simulink model "Closed_loop_DC_motor_speed_control"  (R2024a)
settings: Solver=FixedStepAuto  StartTime=0.0  StopTime=3  RelTol=1e-3
values from neighbouring files (symbols this model uses):
  J = 0.00252    [DC_motor_setting.m]
  Kac = 1 / Kpc    (= 0.066209727553)    [DC_motor_setting.m]
  Kas = 1 / Kps    (= 0.0948585204168)    [DC_motor_setting.m]
  Kic = Ra * wcc    (= 2309.95024633)    [DC_motor_setting.m]
  Kis = Kps * wcs / 5    (= 3746.38945888)    [DC_motor_setting.m]
  Kpc = La * wcc    (= 15.1035208414)    [DC_motor_setting.m]
  Kps = J * wcs / Kt    (= 10.5420155786)    [DC_motor_setting.m]
  Kt = Te_rated / Ia_rated    (= 0.424752712124)    [DC_motor_setting.m]
  La = 1.7e-3    (= 0.0017)    [DC_motor_setting.m]
  Ra = 0.26    [DC_motor_setting.m]
  Te_rated = power_rated / wm_rated    (= 10.6188178031)    [DC_motor_setting.m]
  TL = 1    [DC_motor_setting.m]
  Tsw = 1 / fsw    (= 5e-05)    [DC_motor_setting.m]
  Va_rated = 140    [DC_motor_setting.m]
  Vdc = 200    [DC_motor_setting.m]
libraries: spsDCMachineLib x1, spsDCVoltageSourceLib x1, simulink x1, spsUniversalBridgeLib x1, sps_lib x1
settings Model: Creator=d  LastModifiedBy=d

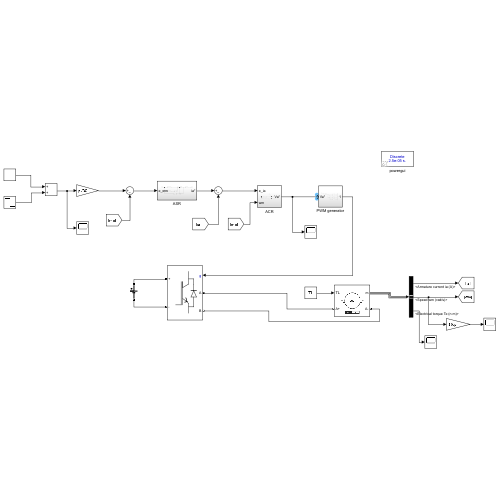
[thumbnail: Simulink's stored preview of the top-level diagram]
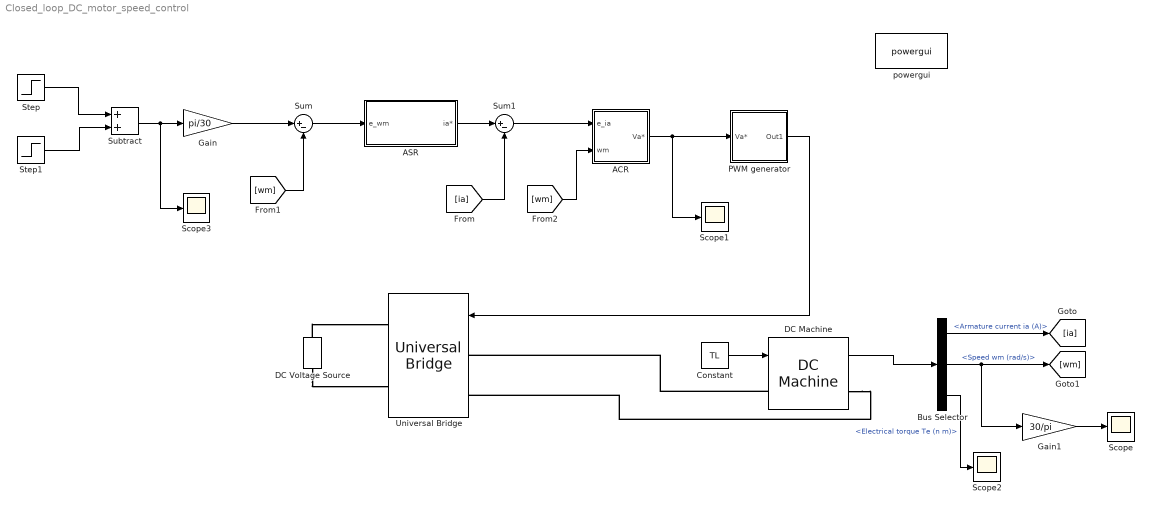
== system Closed_loop_DC_motor_speed_control ==
  ACR : Subsystem
  ASR : Subsystem
  Bus Selector : BusSelector  OutputSignals=Armature current ia (A),Speed wm (rad/s),Electrical torque Te (n m)
  Constant : Constant  Value=TL
  DC Machine : spsDCMachineLib/DC Machine  PresetModel=No  MechanicalLoad=Torque TL  FieldType=Permanent magnet  ShowDetailedParameters=on  MeasurementBus=off  RLa="[ Ra  La]"  RLf="[ 240  120]"  Laf=1.8  MachineConstant=Torque constant (N.m/A)  Ke=1.8  Kt=Kt  J=J  Bm=B  Tf=0  w0=0  Ifinit=1  TsPowergui=0  TsBlock=-1
  DC Voltage Source : spsDCVoltageSourceLib/DC Voltage Source  Amplitude=Vdc  Measurements=None
  Gain : Gain  Gain=pi/30
  Gain1 : Gain  Gain=30/pi
  PWM generator : Subsystem
  Scope{,1..3} (4 alike) : Scope
  Step : Step  After=1000  SampleTime=0
  Step1 : Step  Time=2  After=-2000  SampleTime=0
  Subtract : Sum
  Sum : Sum  Inputs=|+-
  Sum1 : Sum  Inputs=|+-
  Universal Bridge : spsUniversalBridgeLib/Universal Bridge  Arms=2  SnubberResistance=1e5  SnubberCapacitance=inf  Device=IGBT / Diodes  Ron=1e-3  Lon=0  ForwardVoltages="[  0  0  ]"  ForwardVoltage=0  GTOparameters=[ 10e-6 , 20e-6 ]  IGBTparameters=[ 1e-6 , 2e-6 ]  Measurements=None  Measurements_2=None  converterType=Rectifier
  powergui : sps_lib/powergui  Priority=1  SimulationMode=Discrete  SampleTime=Tsw/4  frequency=60  Iterations=50  frequencyindice=0  Pbase=100e6  ErrMax=1e-4  UnitsV=kV  UnitsW=MW  buscounter=0  FunctionMessages=off  echomessages=off  EnableUseOfTLC=off  CurrentSourceSwitches=off  DisableSnubberDevices=off  DisableRonSwitches=off  DisableVfSwitches=off  DisplayEquations=off  AutomaticDiscreteSolvers=off  SolverType=Tustin/Backward Euler (TBE)  Interpol=off  ExternalGateDelay=off  methode=off  Ts=100  x0status=blocks  SPID=on  SwTol=0  HookPort=off  NonlinearTolerance=1e-4  nMaxIteration=100  ContinueOnMaxIteration=off  RestoreLinks=warning  ResistiveCurrentMeasurement=off  Frange=[0:2:500]  Ylog=off  Xlog=on  ShowGrid=off  save=off  variable=ZData  structure=0  ZoomFFT=off  StartTime=0.0  cycles=1  DisplayStyle=1  fundamental=60  FreqAxis=off  MaxFrequency=1000  frequencyindicesteady=1  RmsSteady=1  display=off
  wires:
  Step/1 -> Subtract/1
  Step1/1 -> Subtract/2
  Subtract/1 -> Scope3/1, Gain/1
  Gain/1 -> Sum/1
  Sum/1 -> ASR/1(e_wm)
  ASR/1(ia*) -> Sum1/1
  PWM generator/1(Out1) -> Universal Bridge/1
  Constant/1 -> DC Machine/1
  DC Machine/1 -> Bus Selector/1
  Bus Selector/1 -> [ia]  "<Armature current ia (A)>"
  Bus Selector/2 -> Gain1/1, [wm]  "<Speed wm (rad/s)>"
  [ia] -> Sum1/2
  [wm] -> Sum/2
  Sum1/1 -> ACR/1(e_ia)
  ACR/1(Va*) -> Scope1/1, PWM generator/1(Va*)
  [wm] -> ACR/2(wm)
  Gain1/1 -> Scope/1
  Bus Selector/3 -> Scope2/1  "<Electrical torque Te (n m)>"
  connections:
  DC Voltage Source/RConn1 -- Universal Bridge/RConn1
  DC Voltage Source/LConn1 -- Universal Bridge/RConn2
  DC Machine/RConn1 -- Universal Bridge/LConn2
  DC Machine/LConn1 -- Universal Bridge/LConn1

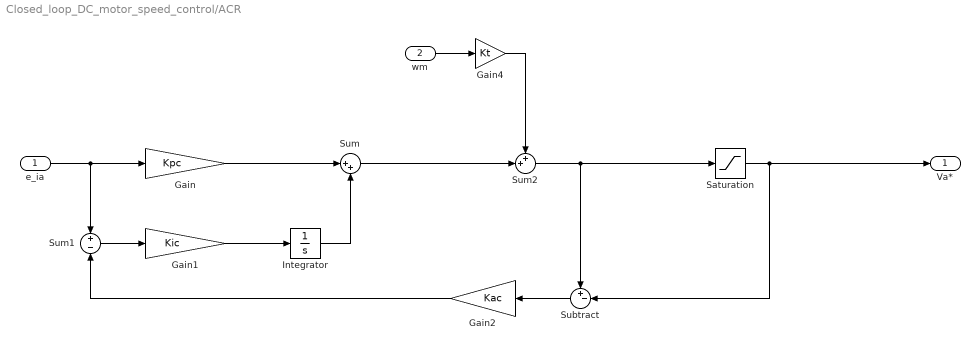
== system Closed_loop_DC_motor_speed_control/ACR ==
  e_ia : Inport
  wm : Inport  Port=2
  Gain : Gain  Gain=Kpc
  Gain1 : Gain  Gain=Kic
  Gain2 : Gain  Gain=Kac
  Gain4 : Gain  Gain=Kt
  Integrator : Integrator
  Saturation : Saturate  UpperLimit=Va_rated  LowerLimit=-Va_rated
  Subtract : Sum  Inputs=+-|
  Sum : Sum  Inputs=|++
  Sum1 : Sum  Inputs=+|-
  Sum2 : Sum  Inputs=++|
  Va* : Outport
  wires:
  Gain2/1 -> Sum1/2
  Sum1/1 -> Gain1/1
  Integrator/1 -> Sum/2
  Saturation/1 -> Va*/1, Subtract/2
  Gain1/1 -> Integrator/1
  e_ia/1 -> Sum1/1, Gain/1
  Gain/1 -> Sum/1
  Subtract/1 -> Gain2/1
  wm/1 -> Gain4/1
  Sum/1 -> Sum2/2
  Sum2/1 -> Subtract/1, Saturation/1
  Gain4/1 -> Sum2/1

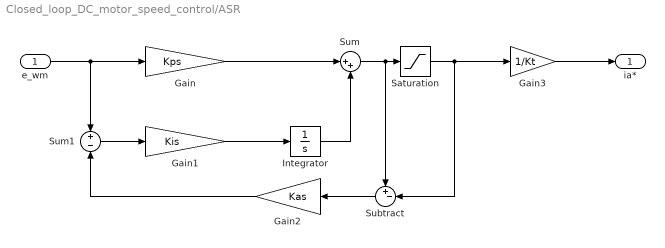
== system Closed_loop_DC_motor_speed_control/ASR ==
  e_wm : Inport
  Gain : Gain  Gain=Kps
  Gain1 : Gain  Gain=Kis
  Gain2 : Gain  Gain=Kas
  Gain3 : Gain  Gain=1/Kt
  Integrator : Integrator
  Saturation : Saturate  UpperLimit=Te_rated  LowerLimit=-Te_rated
  Subtract : Sum  Inputs=+-|
  Sum : Sum  Inputs=|++
  Sum1 : Sum  Inputs=+|-
  ia* : Outport
  wires:
  e_wm/1 -> Sum1/1, Gain/1
  Gain1/1 -> Integrator/1
  Gain/1 -> Sum/1
  Integrator/1 -> Sum/2
  Sum/1 -> Subtract/1, Saturation/1
  Saturation/1 -> Gain3/1, Subtract/2
  Subtract/1 -> Gain2/1
  Sum1/1 -> Gain1/1
  Gain2/1 -> Sum1/2
  Gain3/1 -> ia*/1

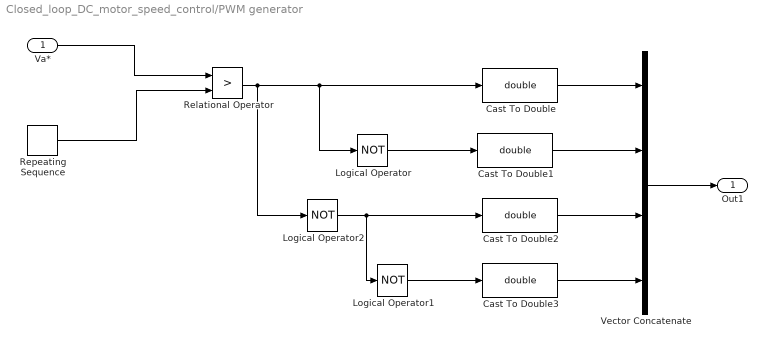
== system Closed_loop_DC_motor_speed_control/PWM generator ==
  Va* : Inport
  Cast To Double{,1..3} (4 alike) : DataTypeConversion  OutDataTypeStr=double  SaturateOnIntegerOverflow=off  RndMeth=Floor
  Logical Operator : Logic  Operator=NOT  AllPortsSameDT=off  OutDataTypeStr=boolean
  Logical Operator1 : Logic  Operator=NOT  AllPortsSameDT=off  OutDataTypeStr=boolean
  Logical Operator2 : Logic  Operator=NOT  AllPortsSameDT=off  OutDataTypeStr=boolean
  Relational Operator : RelationalOperator  Operator=>  OutDataTypeStr=boolean  RndMeth=Simplest  InputSameDT=off
  Repeating Sequence : simulink/Sources/Repeating Sequence  rep_seq_t=[0 0.5*Tsw Tsw]  rep_seq_y=[-Vdc Vdc -Vdc]
  Vector Concatenate : Concatenate  NumInputs=4
  Out1 : Outport
  wires:
  Va*/1 -> Relational Operator/1
  Repeating Sequence/1 -> Relational Operator/2
  Relational Operator/1 -> Logical Operator2/1, Cast To Double/1, Logical Operator/1
  Logical Operator/1 -> Cast To Double1/1
  Logical Operator1/1 -> Cast To Double3/1
  Logical Operator2/1 -> Logical Operator1/1, Cast To Double2/1
  Cast To Double3/1 -> Vector Concatenate/4
  Cast To Double2/1 -> Vector Concatenate/3
  Cast To Double1/1 -> Vector Concatenate/2
  Cast To Double/1 -> Vector Concatenate/1
  Vector Concatenate/1 -> Out1/1
